simulink model "cos"  (R2018b)
settings: Solver=ode4  StartTime=0.0  StopTime=inf  FixedStep=0.01  RelTol=1e-3
undefined symbols (not defined in the file): canChannel
libraries: canlib x7, canmsglib x6
settings Model: Creator=LPA4  LastModifiedBy=User
settings SFSimCC: SimUseLocalCustomCode=off
settings RTWCC: RTWUseLocalCustomCode=off
settings CodeAppCC: StateflowObjectComments=on

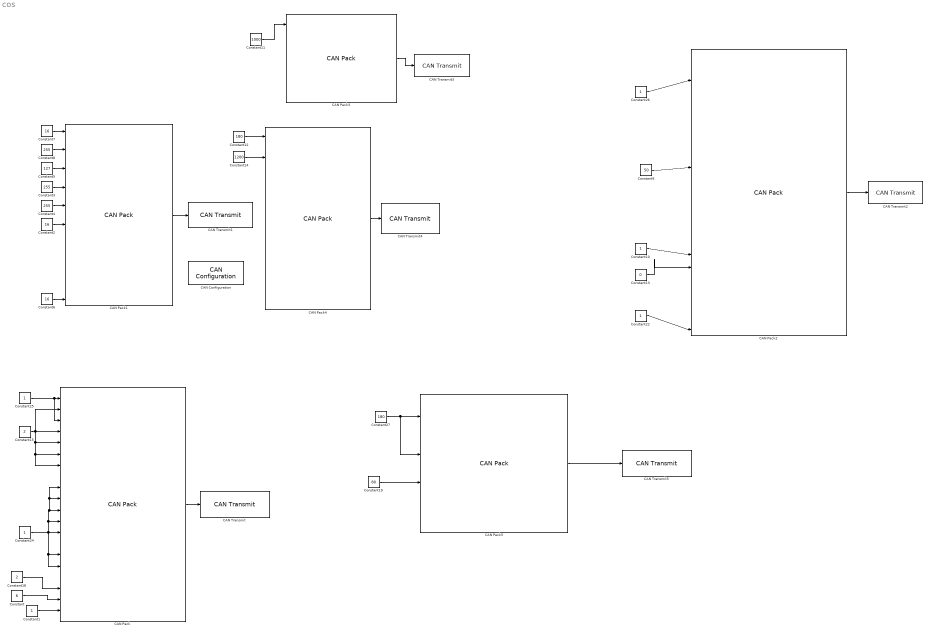
== system cos ==
  CAN Configuration : canlib/CAN Configuration  BlockHandle=4.0001  DeviceMenu=MathWorks Virtual 1 (Channel 1)  Device=Vector CANcardXL 1 (Channel 2)  ObjConstructor=canChannel('Vector', 'CANcardXL 1', 2)  BusSpeed=500000  EnableBitParameters=off  SJW=1  TSEG1=4  TSEG2=3  NSamples=1  AckMode=Normal
      settings: SourceProductName=Vehicle Network Toolbox  SourceProductBaseCode=VN
  CAN Pack : canmsglib/CAN Pack  CANdbFile=C:\Users\LPA4\Desktop\poziomki\database (2).dbc  MsgList=HMIIOM_Disp_01P  MsgName=HMIIOM_Disp_01P  MsgIDType=Extended (29-bit identifier)  MsgIdentifier=285151215  MsgLength=8  SignalInfo=AdBlueLevelLowAlert_cmd$3$3$1$2$1$0$1$0$-Inf$Inf$#CheckAlert_cmd$33$3$1$2$1$0$1$0$-Inf$Inf$#DippedBeamAlert_cmd$15$3$1$2$1$0$1$0$-Inf$Inf$#DirIndicatorLeftAlert_cmd$27$3$1$2$1$0$1$0$-Inf$Inf$#DirIndicatorLtTrailerAlert_cmd$42$3$1$2$1$0$1$0$-Inf$Inf$#DirIndicatorRightAlert_cmd$9$3$1$2$1$0$1$0$-Inf$Inf$#DirIndicatorRtTrailerAlert_cmd$18$3$1$2$1$0$1$0$-Inf$Inf$#EngineMalFunctionAlert_cmd$39$3$1$2$1$0$1$0$-Inf$Inf$#ExtraSpotLampsAlert_cmd$24$3$1$2$1$0$1$0$-Inf$Inf$#FogLightFrontAlert_cmd$45$3$1$2$1$0$1$0$-Inf$Inf$#FogLightRearAlert_cmd$30$3$1$2$1$0$1$0$-Inf$Inf$#FuelLevelLowAlert_cmd$36$3$1$2$1$0$1$0$-Inf$Inf$#LiftAxle1Alert_cmd$6$3$1$2$1$0$1$0$-Inf$Inf$#LiftAxle2Alert_cmd$0$3$1$2$1$0$1$0$-Inf$Inf$#MainBeamAlert_cmd$12$3$1$2$1$0$1$0$-Inf$Inf$#ParkBrakeAlert_cmd$21$3$1$2$1$0$1$0$-Inf$Inf$#PosLightAlert_cmd$48$3$1$2$1$0$1$0$-Inf$Inf$#StopAlert_cmd$51$3$1$2$1$0$1$0$-Inf$Inf$#VehicleMode$54$4$1$2$1$0$1$0$-Inf$Inf$#VehicleMode_UB$58$1$1$2$1$0$1$0$-Inf$Inf$#  NSignals=20  StartBits=str2num('[int32(3);int32(33);int32(15);int32(27);int32(42);int32(9);int32(18);int32(39);int32(24);int32(45);int32(30);int32(36);int32(6);int32(0);int32(12);int32(21);int32(48);int32(51);int32(54);int32(58)]')  SignalSizes=str2num('[int32(3);int32(3);int32(3);int32(3);int32(3);int32(3);int32(3);int32(3);int32(3);int32(3);int32(3);int32(3);int32(3);int32(3);int32(3);int32(3);int32(3);int32(3);int32(4);int32(1)]')  ByteOrders=str2num('[int32(1);int32(1);int32(1);int32(1);int32(1);int32(1);int32(1);int32(1);int32(1);int32(1);int32(1);int32(1);int32(1);int32(1);int32(1);int32(1);int32(1);int32(1);int32(1);int32(1)]')  DataTypes=str2num('[int32(2);int32(2);int32(2);int32(2);int32(2);int32(2);int32(2);int32(2);int32(2);int32(2);int32(2);int32(2);int32(2);int32(2);int32(2);int32(2);int32(2);int32(2);int32(2);int32(2)]')  MultiplexTypes=str2num('[int32(1);int32(1);int32(1);int32(1);int32(1);int32(1);int32(1);int32(1);int32(1);int32(1);int32(1);int32(1);int32(1);int32(1);int32(1);int32(1);int32(1);int32(1);int32(1);int32(1)]')  MultiplexValues=str2num('[double(0);double(0);double(0);double(0);double(0);double(0);double(0);double(0);double(0);double(0);double(0);double(0);double(0);double(0);double(0);double(0);double(0);double(0);double(0);double(0)]')  Factors=str2num('[double(1);double(1);double(1);double(1);double(1);double(1);double(1);double(1);double(1);double(1);double(1);double(1);double(1);double(1);double(1);double(1);double(1);double(1);double(1);double(1)]')  Offsets=str2num('[double(0);double(0);double(0);double(0);double(0);double(0);double(0);double(0);double(0);double(0);double(0);double(0);double(0);double(0);double(0);double(0);double(0);double(0);double(0);double(0)]')  Minimums=str2num('[double(-Inf);double(-Inf);double(-Inf);double(-Inf);double(-Inf);double(-Inf);double(-Inf);double(-Inf);double(-Inf);double(-Inf);double(-Inf);double(-Inf);double(-Inf);double(-Inf);double(-Inf);double(-Inf);double(-Inf);double(-Inf);double(-Inf);double(-Inf)]')  Maximums=str2num('[double(Inf);double(Inf);double(Inf);double(Inf);double(Inf);double(Inf);double(Inf);double(Inf);double(Inf);double(Inf);double(Inf);double(Inf);double(Inf);double(Inf);double(Inf);double(Inf);double(Inf);double(Inf);double(Inf);double(Inf)]')  Remote=off  ApplyMinMax=off  BusOutput=off
      settings: SourceProductName=Simulink Real-Time  SourceProductBaseCode=XP  DataFormat=CANdb specified signals
  CAN Pack1 : canmsglib/CAN Pack  CANdbFile=C:\Users\LPA4\Desktop\poziomki\database (2).dbc  MsgList=HMIIOM_Disp_11P  MsgName=HMIIOM_Disp_11P  MsgIDType=Extended (29-bit identifier)  MsgIdentifier=285192159  MsgLength=8  SignalInfo=BacklightCmd$48$5$1$2$1$0$1$0$-Inf$Inf$#ClusterDispIllumLvlCmd$8$8$1$2$1$0$1$0$0$255$#ContrastLevelCmd$40$7$1$2$1$0$1$0$0$127$#DIDIlluminationLevel_cmd$16$8$1$2$1$0$1$0$0$255$#GaugeIllumLevelCmd$32$8$1$2$1$0$1$0$0$255$#LEDIntensity$53$5$1$2$1$0$1$0$-Inf$Inf$#SIDIlluminationLevel_cmd$24$8$1$2$1$0$1$0$0$255$#SIDOnOff$6$2$1$2$1$0$1$0$-Inf$Inf$#SelectedLanguage_stat$0$6$1$2$1$0$1$0$-Inf$Inf$#TelltaleIntensity$58$5$1$2$1$0$1$0$-Inf$Inf$#  NSignals=10  StartBits=str2num('[int32(48);int32(8);int32(40);int32(16);int32(32);int32(53);int32(24);int32(6);int32(0);int32(58)]')  SignalSizes=str2num('[int32(5);int32(8);int32(7);int32(8);int32(8);int32(5);int32(8);int32(2);int32(6);int32(5)]')  ByteOrders=str2num('[int32(1);int32(1);int32(1);int32(1);int32(1);int32(1);int32(1);int32(1);int32(1);int32(1)]')  DataTypes=str2num('[int32(2);int32(2);int32(2);int32(2);int32(2);int32(2);int32(2);int32(2);int32(2);int32(2)]')  MultiplexTypes=str2num('[int32(1);int32(1);int32(1);int32(1);int32(1);int32(1);int32(1);int32(1);int32(1);int32(1)]')  MultiplexValues=str2num('[double(0);double(0);double(0);double(0);double(0);double(0);double(0);double(0);double(0);double(0)]')  Factors=str2num('[double(1);double(1);double(1);double(1);double(1);double(1);double(1);double(1);double(1);double(1)]')  Offsets=str2num('[double(0);double(0);double(0);double(0);double(0);double(0);double(0);double(0);double(0);double(0)]')  Minimums=str2num('[double(-Inf);double(0);double(0);double(0);double(0);double(-Inf);double(0);double(-Inf);double(-Inf);double(-Inf)]')  Maximums=str2num('[double(Inf);double(255);double(127);double(255);double(255);double(Inf);double(255);double(Inf);double(Inf);double(Inf)]')  Remote=off  ApplyMinMax=off  BusOutput=off
      settings: SourceProductName=Simulink Real-Time  SourceProductBaseCode=XP  DataFormat=CANdb specified signals
  CAN Pack2 : canmsglib/CAN Pack  CANdbFile=C:\Users\LPA4\Desktop\poziomki\database (2).dbc  MsgList=HMIIOM_Disp_03P  MsgName=HMIIOM_Disp_03P  MsgIDType=Extended (29-bit identifier)  MsgIdentifier=285167535  MsgLength=8  SignalInfo=LCDFormattedVehSpdBlink_cmd$29$2$1$2$1$0$1$0$-Inf$Inf$#PresVal_ACCReducedMode$4$2$1$2$1$0$1$0$-Inf$Inf$#PresVal_ACCStatus$12$2$1$2$1$0$1$0$-Inf$Inf$#PresVal_AmbientAirTempUnit$24$2$1$2$1$0$1$0$-Inf$Inf$#PresVal_AuxiliaryBrakesActivat$20$2$1$2$1$0$1$0$-Inf$Inf$#PresVal_AuxiliaryBrakesPos$32$3$1$2$1$0$1$0$-Inf$Inf$#PresVal_CatalystTankLevelLow$18$2$1$2$1$0$1$0$-Inf$Inf$#PresVal_CrossCountryStatus$2$2$1$2$1$0$1$0$-Inf$Inf$#PresVal_EngSpdCtrlStatus$54$2$1$2$1$0$1$0$-Inf$Inf$#PresVal_FuelLevel$56$8$1$2$1$0$4.000000e-01$0$0$102$#PresVal_LowAmbientTempWarning$0$2$1$2$1$0$1$0$-Inf$Inf$#PresVal_LowFuelLevelWrn_stat$14$2$1$2$1$0$1$0$-Inf$Inf$#PresVal_OdometerUnit$8$2$1$2$1$0$1$0$-Inf$Inf$#PresVal_TargetDetected$10$2$1$2$1$0$1$0$-Inf$Inf$#PresVal_TripmeterChoice$16$2$1$2$1$0$1$0$-Inf$Inf$#SIDPresentationMode$50$4$1$2$1$0$1$0$-Inf$Inf$#SeatBeltReminderAlert_cmd$38$3$1$2$1$0$1$0$-Inf$Inf$#VehicleSpeedLCDSpeedUnitCmd$22$2$1$2$1$0$1$0$-Inf$Inf$#ZoningBandsActiveBlueLEDRange1$26$3$1$2$1$0$1$0$-Inf$Inf$#ZoningBandsActiveBlueLEDRange2$47$3$1$2$1$0$1$0$-Inf$Inf$#ZoningBandsActiveGreenLEDRng1$41$3$1$2$1$0$1$0$-Inf$Inf$#ZoningBandsActiveGreenLEDRng2$44$3$1$2$1$0$1$0$-Inf$Inf$#ZoningBandsActiveRedLEDRange1$35$3$1$2$1$0$1$0$-Inf$Inf$#  NSignals=23  StartBits=str2num('[int32(29);int32(4);int32(12);int32(24);int32(20);int32(32);int32(18);int32(2);int32(54);int32(56);int32(0);int32(14);int32(8);int32(10);int32(16);int32(50);int32(38);int32(22);int32(26);int32(47);int32(41);int32(44);int32(35)]')  SignalSizes=str2num('[int32(2);int32(2);int32(2);int32(2);int32(2);int32(3);int32(2);int32(2);int32(2);int32(8);int32(2);int32(2);int32(2);int32(2);int32(2);int32(4);int32(3);int32(2);int32(3);int32(3);int32(3);int32(3);int32(3)]')  ByteOrders=str2num('[int32(1);int32(1);int32(1);int32(1);int32(1);int32(1);int32(1);int32(1);int32(1);int32(1);int32(1);int32(1);int32(1);int32(1);int32(1);int32(1);int32(1);int32(1);int32(1);int32(1);int32(1);int32(1);int32(1)]')  DataTypes=str2num('[int32(2);int32(2);int32(2);int32(2);int32(2);int32(2);int32(2);int32(2);int32(2);int32(2);int32(2);int32(2);int32(2);int32(2);int32(2);int32(2);int32(2);int32(2);int32(2);int32(2);int32(2);int32(2);int32(2)]')  MultiplexTypes=str2num('[int32(1);int32(1);int32(1);int32(1);int32(1);int32(1);int32(1);int32(1);int32(1);int32(1);int32(1);int32(1);int32(1);int32(1);int32(1);int32(1);int32(1);int32(1);int32(1);int32(1);int32(1);int32(1);int32(1)]')  MultiplexValues=str2num('[double(0);double(0);double(0);double(0);double(0);double(0);double(0);double(0);double(0);double(0);double(0);double(0);double(0);double(0);double(0);double(0);double(0);double(0);double(0);double(0);double(0);double(0);double(0)]')  Factors=str2num('[double(1);double(1);double(1);double(1);double(1);double(1);double(1);double(1);double(1);double(4.000000e-01);double(1);double(1);double(1);double(1);double(1);double(1);double(1);double(1);double(1);double(1);double(1);double(1);double(1)]')  Offsets=str2num('[double(0);double(0);double(0);double(0);double(0);double(0);double(0);double(0);double(0);double(0);double(0);double(0);double(0);double(0);double(0);double(0);double(0);double(0);double(0);double(0);double(0);double(0);double(0)]')  Minimums=str2num('[double(-Inf);double(-Inf);double(-Inf);double(-Inf);double(-Inf);double(-Inf);double(-Inf);double(-Inf);double(-Inf);double(0);double(-Inf);double(-Inf);double(-Inf);double(-Inf);double(-Inf);double(-Inf);double(-Inf);double(-Inf);double(-Inf);double(-Inf);double(-Inf);double(-Inf);double(-Inf)]')  Maximums=str2num('[double(Inf);double(Inf);double(Inf);double(Inf);double(Inf);double(Inf);double(Inf);double(Inf);double(Inf);double(102);double(Inf);double(Inf);double(Inf);double(Inf);double(Inf);double(Inf);double(Inf);double(Inf);double(Inf);double(Inf);double(Inf);double(Inf);double(Inf)]')  Remote=off  ApplyMinMax=off  BusOutput=off
      settings: SourceProductName=Simulink Real-Time  SourceProductBaseCode=XP  DataFormat=CANdb specified signals
  CAN Pack3 : canmsglib/CAN Pack  CANdbFile=C:\Users\LPA4\Desktop\poziomki\database (2).dbc  MsgList=HMIIOM_Disp_05P  MsgName=HMIIOM_Disp_05P  MsgIDType=Extended (29-bit identifier)  MsgIdentifier=285183855  MsgLength=8  SignalInfo=PresVal_EngineSpeed$0$16$1$2$1$0$1.250000e-01$0$0$8.191875e+03$#PresVal_TransmSelectedGear$32$16$1$2$1$0$1$0$-Inf$Inf$#PresVal_VehicleSpeed$16$16$1$2$1$0$3.906250e-03$0$0$2.559961e+02$#SpeedometerPSDViewCurrentSpeed$48$16$1$2$1$0$3.906250e-03$0$0$2.559961e+02$#  NSignals=4  StartBits=str2num('[int32(0);int32(32);int32(16);int32(48)]')  SignalSizes=str2num('[int32(16);int32(16);int32(16);int32(16)]')  ByteOrders=str2num('[int32(1);int32(1);int32(1);int32(1)]')  DataTypes=str2num('[int32(2);int32(2);int32(2);int32(2)]')  MultiplexTypes=str2num('[int32(1);int32(1);int32(1);int32(1)]')  MultiplexValues=str2num('[double(0);double(0);double(0);double(0)]')  Factors=str2num('[double(1.250000e-01);double(1);double(3.906250e-03);double(3.906250e-03)]')  Offsets=str2num('[double(0);double(0);double(0);double(0)]')  Minimums=str2num('[double(0);double(-Inf);double(0);double(0)]')  Maximums=str2num('[double(8.191875e+03);double(Inf);double(2.559961e+02);double(2.559961e+02)]')  Remote=off  ApplyMinMax=off  BusOutput=off
      settings: SourceProductName=Simulink Real-Time  SourceProductBaseCode=XP  DataFormat=CANdb specified signals
  CAN Pack4 : canmsglib/CAN Pack  CANdbFile=C:\Users\LPA4\Desktop\poziomki\database (2).dbc  MsgList=HMIIOM_Disp_04P  MsgName=HMIIOM_Disp_04P  MsgIDType=Extended (29-bit identifier)  MsgIdentifier=285175695  MsgLength=8  SignalInfo=FormatedVehicleSpeed$0$8$1$2$1$0$1$0$0$255$#PresVal_AirPressure$32$8$1$2$1$0$8$0$0$2040$#PresVal_AmbientAirTemperature$40$9$1$2$1$0$5.000000e-01$-60$-60$1.955000e+02$#PresVal_AvailGearsHigherRatio$56$4$1$2$1$0$1$0$0$15$#PresVal_AvailGearsLowerRatio$60$4$1$2$1$0$1$0$0$15$#PresVal_CatalystTankLevel$8$8$1$2$1$0$4.000000e-01$0$0$102$#PresVal_ClockHours$16$8$1$2$1$0$1$0$0$255$#PresVal_ClockMinutes$24$8$1$2$1$0$1$0$0$255$#PresVal_ClockPeriod$51$3$1$2$1$0$1$0$-Inf$Inf$#  NSignals=9  StartBits=str2num('[int32(0);int32(32);int32(40);int32(56);int32(60);int32(8);int32(16);int32(24);int32(51)]')  SignalSizes=str2num('[int32(8);int32(8);int32(9);int32(4);int32(4);int32(8);int32(8);int32(8);int32(3)]')  ByteOrders=str2num('[int32(1);int32(1);int32(1);int32(1);int32(1);int32(1);int32(1);int32(1);int32(1)]')  DataTypes=str2num('[int32(2);int32(2);int32(2);int32(2);int32(2);int32(2);int32(2);int32(2);int32(2)]')  MultiplexTypes=str2num('[int32(1);int32(1);int32(1);int32(1);int32(1);int32(1);int32(1);int32(1);int32(1)]')  MultiplexValues=str2num('[double(0);double(0);double(0);double(0);double(0);double(0);double(0);double(0);double(0)]')  Factors=str2num('[double(1);double(8);double(5.000000e-01);double(1);double(1);double(4.000000e-01);double(1);double(1);double(1)]')  Offsets=str2num('[double(0);double(0);double(-60);double(0);double(0);double(0);double(0);double(0);double(0)]')  Minimums=str2num('[double(0);double(0);double(-60);double(0);double(0);double(0);double(0);double(0);double(-Inf)]')  Maximums=str2num('[double(255);double(2040);double(1.955000e+02);double(15);double(15);double(102);double(255);double(255);double(Inf)]')  Remote=off  ApplyMinMax=off  BusOutput=off
      settings: SourceProductName=Simulink Real-Time  SourceProductBaseCode=XP  DataFormat=CANdb specified signals
  CAN Pack5 : canmsglib/CAN Pack  CANdbFile=C:\Users\LPA4\Desktop\poziomki\database (2).dbc  MsgList=HMIIOM_Disp_08P  MsgName=HMIIOM_Disp_08P  MsgIDType=Extended (29-bit identifier)  MsgIdentifier=285192111  MsgLength=8  SignalInfo=PresValReqTimeGap$56$3$1$2$1$0$1$0$-Inf$Inf$#PresVal_ASLActiveStatus$18$2$1$2$1$0$1$0$-Inf$Inf$#PresVal_ASLSetSpeed$0$8$1$2$1$0$1$0$0$255$#PresVal_ASLSpeedBlinkCmd$32$2$1$2$1$0$1$0$-Inf$Inf$#PresVal_CCActiveStatus$20$2$1$2$1$0$1$0$-Inf$Inf$#PresVal_CCEnabledStatus$22$2$1$2$1$0$1$0$-Inf$Inf$#PresVal_CCSetSpeed$8$8$1$2$1$0$1$0$0$255$#PresVal_CCSpeedBlinkCmd$34$2$1$2$1$0$1$0$-Inf$Inf$#PresVal_CCSpeedInactive$36$2$1$2$1$0$1$0$-Inf$Inf$#PresVal_CoolantTemp$24$8$1$2$1$0$1$-40$-40$215$#PresVal_CoolantTempHigh$38$2$1$2$1$0$1$0$-Inf$Inf$#PresVal_EngineCoolantTemp$40$8$1$2$1$0$4.000000e-01$0$0$102$#PresVal_GearLeverModeASCII$48$8$1$2$1$0$1$0$-Inf$Inf$#PresVal_GearLeverModeBlink$16$2$1$2$1$0$1$0$-Inf$Inf$#PresVal_GearLeverModeFrame$59$2$1$2$1$0$1$0$-Inf$Inf$#  NSignals=15  StartBits=str2num('[int32(56);int32(18);int32(0);int32(32);int32(20);int32(22);int32(8);int32(34);int32(36);int32(24);int32(38);int32(40);int32(48);int32(16);int32(59)]')  SignalSizes=str2num('[int32(3);int32(2);int32(8);int32(2);int32(2);int32(2);int32(8);int32(2);int32(2);int32(8);int32(2);int32(8);int32(8);int32(2);int32(2)]')  ByteOrders=str2num('[int32(1);int32(1);int32(1);int32(1);int32(1);int32(1);int32(1);int32(1);int32(1);int32(1);int32(1);int32(1);int32(1);int32(1);int32(1)]')  DataTypes=str2num('[int32(2);int32(2);int32(2);int32(2);int32(2);int32(2);int32(2);int32(2);int32(2);int32(2);int32(2);int32(2);int32(2);int32(2);int32(2)]')  MultiplexTypes=str2num('[int32(1);int32(1);int32(1);int32(1);int32(1);int32(1);int32(1);int32(1);int32(1);int32(1);int32(1);int32(1);int32(1);int32(1);int32(1)]')  MultiplexValues=str2num('[double(0);double(0);double(0);double(0);double(0);double(0);double(0);double(0);double(0);double(0);double(0);double(0);double(0);double(0);double(0)]')  Factors=str2num('[double(1);double(1);double(1);double(1);double(1);double(1);double(1);double(1);double(1);double(1);double(1);double(4.000000e-01);double(1);double(1);double(1)]')  Offsets=str2num('[double(0);double(0);double(0);double(0);double(0);double(0);double(0);double(0);double(0);double(-40);double(0);double(0);double(0);double(0);double(0)]')  Minimums=str2num('[double(-Inf);double(-Inf);double(0);double(-Inf);double(-Inf);double(-Inf);double(0);double(-Inf);double(-Inf);double(-40);double(-Inf);double(0);double(-Inf);double(-Inf);double(-Inf)]')  Maximums=str2num('[double(Inf);double(Inf);double(255);double(Inf);double(Inf);double(Inf);double(255);double(Inf);double(Inf);double(215);double(Inf);double(102);double(Inf);double(Inf);double(Inf)]')  Remote=off  ApplyMinMax=off  BusOutput=off
      settings: SourceProductName=Simulink Real-Time  SourceProductBaseCode=XP  DataFormat=CANdb specified signals
  CAN Transmit : canlib/CAN Transmit  BlockHandle=11.0001  DeviceMenu=MathWorks Virtual 1 (Channel 1)  Device=Vector CANcardXL 1 (Channel 2)  ObjConstructor=canChannel('Vector', 'CANcardXL 1', 2)  EnablePeriodicTransmit=on  MessagePeriod=0.01
      settings: SourceProductName=Vehicle Network Toolbox  SourceProductBaseCode=VN
  CAN Transmit1 : canlib/CAN Transmit  BlockHandle=12.0001  DeviceMenu=MathWorks Virtual 1 (Channel 1)  Device=Vector CANcardXL 1 (Channel 2)  ObjConstructor=canChannel('Vector', 'CANcardXL 1', 2)  EnablePeriodicTransmit=on  MessagePeriod=0.01
      settings: SourceProductName=Vehicle Network Toolbox  SourceProductBaseCode=VN
  CAN Transmit2 : canlib/CAN Transmit  BlockHandle=13.0001  DeviceMenu=MathWorks Virtual 1 (Channel 1)  Device=Vector CANcardXL 1 (Channel 2)  ObjConstructor=canChannel('Vector', 'CANcardXL 1', 2)  EnablePeriodicTransmit=on  MessagePeriod=0.01
      settings: SourceProductName=Vehicle Network Toolbox  SourceProductBaseCode=VN
  CAN Transmit3 : canlib/CAN Transmit  BlockHandle=14.0001  DeviceMenu=MathWorks Virtual 1 (Channel 1)  Device=Vector CANcardXL 1 (Channel 2)  ObjConstructor=canChannel('Vector', 'CANcardXL 1', 2)  EnablePeriodicTransmit=on  MessagePeriod=0.01
      settings: SourceProductName=Vehicle Network Toolbox  SourceProductBaseCode=VN
  CAN Transmit4 : canlib/CAN Transmit  BlockHandle=15.0001  DeviceMenu=MathWorks Virtual 1 (Channel 1)  Device=Vector CANcardXL 1 (Channel 2)  ObjConstructor=canChannel('Vector', 'CANcardXL 1', 2)  EnablePeriodicTransmit=on  MessagePeriod=0.01
      settings: SourceProductName=Vehicle Network Toolbox  SourceProductBaseCode=VN
  CAN Transmit5 : canlib/CAN Transmit  BlockHandle=16.0001  DeviceMenu=MathWorks Virtual 1 (Channel 1)  Device=Vector CANcardXL 1 (Channel 2)  ObjConstructor=canChannel('Vector', 'CANcardXL 1', 2)  EnablePeriodicTransmit=on  MessagePeriod=0.01
      settings: SourceProductName=Vehicle Network Toolbox  SourceProductBaseCode=VN
  Constant : Constant  Value=6
  Constant{1,10,22,24..26} (6 alike) : Constant
  Constant11 : Constant  Value=1000
  Constant12 : Constant  Value=180
  Constant13 : Constant  Value=0
  Constant14 : Constant  Value=1200
  Constant15 : Constant  Value=2
  Constant18 : Constant  Value=2
  Constant19 : Constant  Value=80
  Constant2 : Constant  Value=16
  Constant27 : Constant  Value=180
  Constant3 : Constant  Value=255
  Constant4 : Constant  Value=255
  Constant5 : Constant  Value=127
  Constant6 : Constant  Value=16
  Constant7 : Constant  Value=16
  Constant8 : Constant  Value=255
  Constant9 : Constant  Value=50
  wires:
  Constant/1 -> CAN Pack/19
  Constant1/1 -> CAN Pack/20
  Constant2/1 -> CAN Pack1/6
  Constant3/1 -> CAN Pack1/4
  Constant4/1 -> CAN Pack1/5
  Constant5/1 -> CAN Pack1/3
  Constant6/1 -> CAN Pack1/10
  Constant7/1 -> CAN Pack1/1
  Constant8/1 -> CAN Pack1/2
  CAN Pack/1 -> CAN Transmit/1
  CAN Pack1/1 -> CAN Transmit1/1
  Constant9/1 -> CAN Pack2/10
  CAN Pack2/1 -> CAN Transmit2/1
  Constant10/1 -> CAN Pack2/17
  Constant11/1 -> CAN Pack3/1
  CAN Pack3/1 -> CAN Transmit3/1
  CAN Pack4/1 -> CAN Transmit4/1
  Constant12/1 -> CAN Pack4/1
  Constant13/1 -> CAN Pack2/18
  Constant14/1 -> CAN Pack4/2
  Constant24/1 -> CAN Pack/16, CAN Pack/15, CAN Pack/11, CAN Pack/9, CAN Pack/10, CAN Pack/12, CAN Pack/13
  Constant18/1 -> CAN Pack/18
  Constant19/1 -> CAN Pack5/10
  CAN Pack5/1 -> CAN Transmit5/1
  Constant15/1 -> CAN Pack/7, CAN Pack/6, CAN Pack/5, CAN Pack/2, CAN Pack/4
  Constant22/1 -> CAN Pack2/23
  Constant25/1 -> CAN Pack/3, CAN Pack/1
  Constant26/1 -> CAN Pack2/3
  Constant27/1 -> CAN Pack5/7, CAN Pack5/3
